simulink model "examples_of_switch_block"  (R2021a)
settings: Solver=VariableStepAuto  StartTime=0.0  StopTime=10  MaxStep=1e-3  RelTol=1e-3
settings Model: Creator=YasserNet  LastModifiedBy=YasserNet

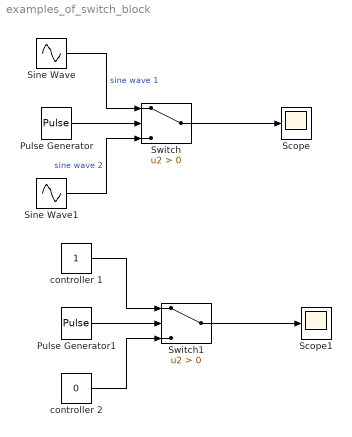
== system examples_of_switch_block ==
  Pulse Generator : DiscretePulseGenerator  PulseType=Time based  Period=1  PulseWidth=50
  Pulse Generator1 : DiscretePulseGenerator  PulseType=Time based  Period=1  PulseWidth=25
  Scope : Scope
  Scope1 : Scope
  Sine Wave : Sin  SampleTime=0
  Sine Wave1 : Sin  Phase=-pi  SampleTime=0
  Switch : Switch  Criteria=u2 > Threshold
  Switch1 : Switch  Criteria=u2 > Threshold
  controller 1 : Constant
  controller 2 : Constant  Value=0
  wires:
  Switch/1 -> Scope/1
  Pulse Generator/1 -> Switch/2
  Sine Wave/1 -> Switch/1  "sine wave 1"
  Sine Wave1/1 -> Switch/3  "sine wave 2"
  Switch1/1 -> Scope1/1
  Pulse Generator1/1 -> Switch1/2
  controller 1/1 -> Switch1/1
  controller 2/1 -> Switch1/3
